simulink model "Cuk_cevirici"  (R2024b)
settings: Solver=ode23tb  StartTime=0.0  StopTime=0.2  RelTol=1e-3
libraries: spsMeanLib x10, spsSeriesRLCBranchLib x10, spsCurrentMeasurementLib x6, spsVoltageMeasurementLib x4, spsDCVoltageSourceLib x2, spsDiodeLib x2, spsGroundLib x2, spsIGBTLib x2, sps_lib x1
settings Model: Creator=m_pek  LastModifiedBy=m_pek

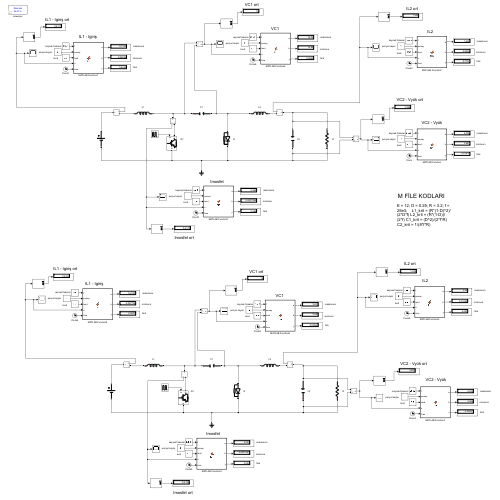
[thumbnail: Simulink's stored preview of the top-level diagram]
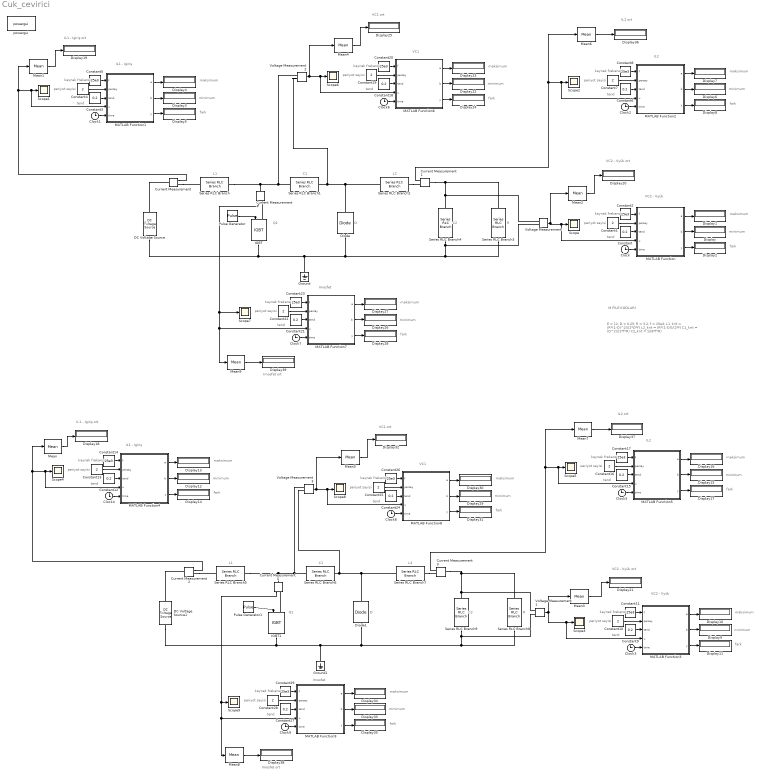
== system Cuk_cevirici ==
  note: M FİLE KODLARI
  note: E = 12; D = 0.25; R = 3.2; f = 25e3; L1_krit = (R*(1-D)^2)/(2*D*f) L2_krit = (R*(1-D))/(2*f) C1_krit = (D^2)/(2*f*R) C2_krit = 1/(8*f*R)
  note: L1
  note: C1
  note: L2
  note: C2
  note: R
  note: D
  note: Q1
  note: E
  note: minimum
  note: kaynak frekansi
  note: fark
  note: tend
  note: periyot sayisi
  note: maksimum
  note: minimum
  note: kaynak frekansi
  note: fark
  note: tend
  note: periyot sayisi
  note: maksimum
  note: minimum
  note: kaynak frekansi
  note: fark
  note: tend
  note: periyot sayisi
  note: maksimum
  note: L1
  note: C1
  note: L2
  note: C2
  note: R
  note: D
  note: Q1
  note: E
  note: minimum
  note: kaynak frekansi
  note: fark
  note: tend
  note: periyot sayisi
  note: maksimum
  note: minimum
  note: kaynak frekansi
  note: fark
  note: tend
  note: periyot sayisi
  note: maksimum
  note: minimum
  note: kaynak frekansi
  note: fark
  note: tend
  note: periyot sayisi
  note: maksimum
  note: VC2 - Vyük ort
  note: IL1 - Igiriş
  note: minimum
  note: kaynak frekansi
  note: fark
  note: tend
  note: periyot sayisi
  note: maksimum
  note: VC1 ort
  note: minimum
  note: kaynak frekansi
  note: fark
  note: tend
  note: periyot sayisi
  note: maksimum
  note: Imosfet
  note: IL1 - Igiriş ort
  note: IL1 - Igiriş ort
  note: IL2
  note: IL2
  note: minimum
  note: kaynak frekansi
  note: fark
  note: tend
  note: periyot sayisi
  note: maksimum
  note: VC1 ort
  note: minimum
  note: kaynak frekansi
  note: fark
  note: tend
  note: periyot sayisi
  note: maksimum
  note: Imosfet
  note: VC2 - Vyük ort
  note: IL2 ort
  note: VC1
  note: VC2 - Vyük
  note: IL2 ort
  note: VC2 - Vyük
  note: IL1 - Igiriş
  note: VC1
  note: Imosfet ort
  note: Imosfet ort
  Clock{,1..9} (10 alike) : Clock
      settings: Decimation=100
  Constant{,3,6,9,12,15,18,21,24,27} (10 alike) : Constant  Value=0.2  SampleTime=0
  Constant{1,4,7,10,13,16,19,22,25,28} (10 alike) : Constant  Value=2  SampleTime=0
  Constant{2,5,8,11,14,17,20,23,26,29} (10 alike) : Constant  Value=25e3  SampleTime=0
  Current Measurement{,1..5} (6 alike) : spsCurrentMeasurementLib/Current Measurement  PhasorSimulation=off  OutputType=Complex  PSBequivalent=0
  DC Voltage Source : spsDCVoltageSourceLib/DC Voltage Source  Amplitude=12  Measurements=None
  DC Voltage Source1 : spsDCVoltageSourceLib/DC Voltage Source  Amplitude=12  Measurements=None
  Diode : spsDiodeLib/Diode  Ron=0.0001  Lon=0  Vf=0.001  IC=0  UseSnubber=0  Rs=5000  Cs=250e-6  Measurements=off
  Diode1 : spsDiodeLib/Diode  Ron=0.0001  Lon=0  Vf=0.001  IC=0  UseSnubber=0  Rs=5000  Cs=250e-6  Measurements=off
  Display{,1..39} (40 alike) : Display
  Ground : spsGroundLib/Ground  LConnTagsString=a
  Ground1 : spsGroundLib/Ground  LConnTagsString=a
  IGBT : spsIGBTLib/IGBT  Ron=0.000001  Lon=0  Vf=0.00001  Tf=1e-6  Tt=2e-6  IC=0  Rs=1e5  Cs=inf  Measurements=off
  IGBT1 : spsIGBTLib/IGBT  Ron=0.000001  Lon=0  Vf=0.00001  Tf=1e-6  Tt=2e-6  IC=0  Rs=1e5  Cs=inf  Measurements=off
  MATLAB Function : MATLAB Function  TreatAsAtomicUnit=on
  MATLAB Function1 : MATLAB Function  TreatAsAtomicUnit=on
  MATLAB Function2 : MATLAB Function  TreatAsAtomicUnit=on
  MATLAB Function3 : MATLAB Function  TreatAsAtomicUnit=on
  MATLAB Function4 : MATLAB Function  TreatAsAtomicUnit=on
  MATLAB Function5 : MATLAB Function  TreatAsAtomicUnit=on
  MATLAB Function6 : MATLAB Function  TreatAsAtomicUnit=on
  MATLAB Function7 : MATLAB Function  TreatAsAtomicUnit=on
  MATLAB Function8 : MATLAB Function  TreatAsAtomicUnit=on
  MATLAB Function9 : MATLAB Function  TreatAsAtomicUnit=on
  Mean{,1..9} (10 alike) : spsMeanLib/Mean  Freq=25e3  Vinit=0  Ts=0
  Pulse Generator : DiscretePulseGenerator  PulseType=Time based  Period=0.00004  PulseWidth=25  VectorParams1D=off
  Pulse Generator1 : DiscretePulseGenerator  PulseType=Time based  Period=0.00004  PulseWidth=25  VectorParams1D=off
  Scope{,1..9} (10 alike) : Scope
  Series RLC Branch : spsSeriesRLCBranchLib/Series RLC Branch  LConnTagsString=__new0  RConnTagsString=__new0  BranchType=L  Resistance=1  Inductance=180e-6  SetiL0=off  InitialCurrent=0  Capacitance=1e-6  Setx0=off  InitialVoltage=0  Measurements=None
  Series RLC Branch1 : spsSeriesRLCBranchLib/Series RLC Branch  LConnTagsString=__new0  RConnTagsString=__new0  BranchType=C  Resistance=1  Inductance=1e-3  SetiL0=off  InitialCurrent=0  Capacitance=200e-6  Setx0=off  InitialVoltage=0  Measurements=None
  Series RLC Branch2 : spsSeriesRLCBranchLib/Series RLC Branch  LConnTagsString=__new0  RConnTagsString=__new0  BranchType=L  Resistance=1  Inductance=150e-6  SetiL0=off  InitialCurrent=0  Capacitance=1e-6  Setx0=off  InitialVoltage=0  Measurements=None
  Series RLC Branch3 : spsSeriesRLCBranchLib/Series RLC Branch  LConnTagsString=__new0  RConnTagsString=__new0  BranchType=R  Resistance=3.2  Inductance=1e-3  SetiL0=off  InitialCurrent=0  Capacitance=1e-6  Setx0=off  InitialVoltage=0  Measurements=None
  Series RLC Branch4 : spsSeriesRLCBranchLib/Series RLC Branch  LConnTagsString=__new0  RConnTagsString=__new0  BranchType=C  Resistance=1  Inductance=1e-3  SetiL0=off  InitialCurrent=0  Capacitance=220e-6  Setx0=off  InitialVoltage=0  Measurements=None
  Series RLC Branch5 : spsSeriesRLCBranchLib/Series RLC Branch  LConnTagsString=__new0  RConnTagsString=__new0  BranchType=L  Resistance=1  Inductance=1.4400e-04  SetiL0=off  InitialCurrent=0  Capacitance=1e-6  Setx0=off  InitialVoltage=0  Measurements=None
  Series RLC Branch6 : spsSeriesRLCBranchLib/Series RLC Branch  LConnTagsString=__new0  RConnTagsString=__new0  BranchType=C  Resistance=1  Inductance=1e-3  SetiL0=off  InitialCurrent=0  Capacitance=200e-6  Setx0=off  InitialVoltage=0  Measurements=None
  Series RLC Branch7 : spsSeriesRLCBranchLib/Series RLC Branch  LConnTagsString=__new0  RConnTagsString=__new0  BranchType=L  Resistance=1  Inductance=4.8000e-05  SetiL0=off  InitialCurrent=0  Capacitance=1e-6  Setx0=off  InitialVoltage=0  Measurements=None
  Series RLC Branch8 : spsSeriesRLCBranchLib/Series RLC Branch  LConnTagsString=__new0  RConnTagsString=__new0  BranchType=R  Resistance=3.2  Inductance=1e-3  SetiL0=off  InitialCurrent=0  Capacitance=1e-6  Setx0=off  InitialVoltage=0  Measurements=None
  Series RLC Branch9 : spsSeriesRLCBranchLib/Series RLC Branch  LConnTagsString=__new0  RConnTagsString=__new0  BranchType=C  Resistance=1  Inductance=1e-3  SetiL0=off  InitialCurrent=0  Capacitance=220e-6  Setx0=off  InitialVoltage=0  Measurements=None
  Voltage Measurement{,1..3} (4 alike) : spsVoltageMeasurementLib/Voltage Measurement  PhasorSimulation=off  OutputType=Complex  PSBequivalent=0
  powergui : sps_lib/powergui  Priority=1  SimulationMode=Discrete  SampleTime=50e-8  frequency=60  Iterations=50  frequencyindice=0  Pbase=100e6  ErrMax=1e-4  UnitsV=kV  UnitsW=MW  buscounter=0  FunctionMessages=off  echomessages=off  EnableUseOfTLC=off  CurrentSourceSwitches=off  DisableSnubberDevices=off  DisableRonSwitches=off  DisableVfSwitches=off  DisplayEquations=off  AutomaticDiscreteSolvers=off  SolverType=Tustin/Backward Euler (TBE)  Interpol=off  ExternalGateDelay=off  methode=off  Ts=100  x0status=zero  SPID=on  SwTol=0  HookPort=off  NonlinearTolerance=1e-4  nMaxIteration=100  ContinueOnMaxIteration=off  RestoreLinks=warning  ResistiveCurrentMeasurement=off  Frange=[0:2:500]  Ylog=off  Xlog=on  ShowGrid=off  save=off  variable=ZData  structure=0  ZoomFFT=off  StartTime=0.0  cycles=1  DisplayStyle=1  fundamental=60  FreqAxis=off  MaxFrequency=1000  frequencyindicesteady=1  RmsSteady=1  display=off
  wires:
  Pulse Generator/1 -> IGBT/1
  MATLAB Function/3(y) -> Display2/1
  MATLAB Function/2(b) -> Display/1
  Clock/1 -> MATLAB Function/5(time)
  Constant/1 -> MATLAB Function/3(tend)
  Constant2/1 -> MATLAB Function/1(f)
  MATLAB Function/1(a) -> Display1/1
  Constant1/1 -> MATLAB Function/2(persay)
  Constant4/1 -> MATLAB Function1/2(persay)
  MATLAB Function1/1(a) -> Display4/1
  Constant5/1 -> MATLAB Function1/1(f)
  Constant3/1 -> MATLAB Function1/3(tend)
  Current Measurement/1 -> Mean1/1, Scope1/1, MATLAB Function1/4(u)
  Clock1/1 -> MATLAB Function1/5(time)
  MATLAB Function1/2(b) -> Display3/1
  MATLAB Function1/3(y) -> Display5/1
  MATLAB Function2/3(y) -> Display8/1
  MATLAB Function2/2(b) -> Display6/1
  Clock2/1 -> MATLAB Function2/5(time)
  Current Measurement1/1 -> Mean6/1, MATLAB Function2/4(u), Scope2/1
  Constant6/1 -> MATLAB Function2/3(tend)
  Constant8/1 -> MATLAB Function2/1(f)
  MATLAB Function2/1(a) -> Display7/1
  Constant7/1 -> MATLAB Function2/2(persay)
  Constant16/1 -> MATLAB Function5/2(persay)
  MATLAB Function5/1(a) -> Display16/1
  Constant17/1 -> MATLAB Function5/1(f)
  Constant15/1 -> MATLAB Function5/3(tend)
  Clock5/1 -> MATLAB Function5/5(time)
  MATLAB Function5/2(b) -> Display15/1
  MATLAB Function5/3(y) -> Display17/1
  MATLAB Function4/3(y) -> Display14/1
  MATLAB Function4/2(b) -> Display12/1
  Clock4/1 -> MATLAB Function4/5(time)
  Current Measurement2/1 -> Mean/1, MATLAB Function4/4(u), Scope4/1
  Constant12/1 -> MATLAB Function4/3(tend)
  Constant14/1 -> MATLAB Function4/1(f)
  MATLAB Function4/1(a) -> Display13/1
  Constant13/1 -> MATLAB Function4/2(persay)
  Constant10/1 -> MATLAB Function3/2(persay)
  MATLAB Function3/1(a) -> Display10/1
  Constant11/1 -> MATLAB Function3/1(f)
  Constant9/1 -> MATLAB Function3/3(tend)
  Clock3/1 -> MATLAB Function3/5(time)
  MATLAB Function3/2(b) -> Display9/1
  MATLAB Function3/3(y) -> Display11/1
  Pulse Generator1/1 -> IGBT1/1
  Mean/1 -> Display18/1
  Mean1/1 -> Display19/1
  Mean2/1 -> Display20/1
  Voltage Measurement/1 -> MATLAB Function/4(u), Scope/1, Mean2/1
  Voltage Measurement1/1 -> Mean3/1, Scope3/1, MATLAB Function3/4(u)
  Mean3/1 -> Display21/1
  Voltage Measurement2/1 -> Scope6/1, MATLAB Function6/4(u), Mean4/1
  Mean4/1 -> Display25/1
  Constant19/1 -> MATLAB Function6/2(persay)
  MATLAB Function6/1(a) -> Display23/1
  Constant20/1 -> MATLAB Function6/1(f)
  Constant18/1 -> MATLAB Function6/3(tend)
  Clock6/1 -> MATLAB Function6/5(time)
  MATLAB Function6/2(b) -> Display22/1
  MATLAB Function6/3(y) -> Display24/1
  Constant22/1 -> MATLAB Function7/2(persay)
  MATLAB Function7/1(a) -> Display27/1
  Constant23/1 -> MATLAB Function7/1(f)
  Constant21/1 -> MATLAB Function7/3(tend)
  Clock7/1 -> MATLAB Function7/5(time)
  MATLAB Function7/2(b) -> Display26/1
  MATLAB Function7/3(y) -> Display28/1
  MATLAB Function8/3(y) -> Display31/1
  MATLAB Function8/2(b) -> Display29/1
  Clock8/1 -> MATLAB Function8/5(time)
  Constant24/1 -> MATLAB Function8/3(tend)
  Constant26/1 -> MATLAB Function8/1(f)
  MATLAB Function8/1(a) -> Display30/1
  Constant25/1 -> MATLAB Function8/2(persay)
  Mean5/1 -> Display32/1
  Voltage Measurement3/1 -> Mean5/1, MATLAB Function8/4(u), Scope8/1
  Current Measurement5/1 -> Mean8/1, MATLAB Function9/4(u), Scope9/1
  MATLAB Function9/3(y) -> Display35/1
  MATLAB Function9/2(b) -> Display33/1
  Clock9/1 -> MATLAB Function9/5(time)
  Constant27/1 -> MATLAB Function9/3(tend)
  Constant29/1 -> MATLAB Function9/1(f)
  MATLAB Function9/1(a) -> Display34/1
  Constant28/1 -> MATLAB Function9/2(persay)
  Mean6/1 -> Display36/1
  Mean7/1 -> Display37/1
  Current Measurement3/1 -> Mean7/1, Scope5/1, MATLAB Function5/4(u)
  Mean8/1 -> Display38/1
  Mean9/1 -> Display39/1
  Current Measurement4/1 -> Scope7/1, MATLAB Function7/4(u), Mean9/1
  connections:
  IGBT/LConn1 -- Current Measurement4/RConn1
  Series RLC Branch2/RConn1 -- Diode/LConn1 -- Voltage Measurement2/LConn2 -- Series RLC Branch1/RConn1
  Current Measurement1/LConn1 -- Voltage Measurement/LConn2 -- Series RLC Branch4/RConn1 -- Series RLC Branch3/RConn1
  DC Voltage Source/LConn1 -- Series RLC Branch4/LConn1 -- Voltage Measurement/LConn1 -- Series RLC Branch3/LConn1 -- Diode/RConn1 -- Ground/LConn1 -- IGBT/RConn1
  DC Voltage Source/RConn1 -- Current Measurement/LConn1
  Current Measurement/RConn1 -- Series RLC Branch/LConn1
  Series RLC Branch2/LConn1 -- Current Measurement1/RConn1
  Series RLC Branch5/RConn1 -- Voltage Measurement3/LConn1 -- Series RLC Branch6/LConn1 -- Current Measurement5/LConn1
  Series RLC Branch7/RConn1 -- Voltage Measurement3/LConn2 -- Series RLC Branch6/RConn1 -- Diode1/LConn1
  Series RLC Branch8/RConn1 -- Current Measurement3/LConn1 -- Voltage Measurement1/LConn2 -- Series RLC Branch9/RConn1
  DC Voltage Source1/LConn1 -- IGBT1/RConn1 -- Ground1/LConn1 -- Diode1/RConn1 -- Voltage Measurement1/LConn1 -- Series RLC Branch9/LConn1 -- Series RLC Branch8/LConn1
  Series RLC Branch7/LConn1 -- Current Measurement3/RConn1
  DC Voltage Source1/RConn1 -- Current Measurement2/LConn1
  Current Measurement2/RConn1 -- Series RLC Branch5/LConn1
  Current Measurement4/LConn1 -- Series RLC Branch/RConn1 -- Voltage Measurement2/LConn1 -- Series RLC Branch1/LConn1
  IGBT1/LConn1 -- Current Measurement5/RConn1

== matlab function Cuk_cevirici/MATLAB Function7 ==
  settings: updateMethod=DISCRETE  sampleTime=50e-8
  data: a output; b output; f input; persay input; tend input; u input; y output; time input
function [a,b,y] = fcn(f,persay,tend,u,time)
% persistent değişken; değişken değerini kalıcı olarak tutar ve direk atama
% yapılmadıkça değişmez. Normal değişkenler fonksiyonun her yenilenme 
% durumunda sıfırlanırken, persistent değişkeni, kalıcı olması sebebiyle,
% bir önceki değeri tutabilme yeteneğine sahiptir. 
% Bu da bize bir önceki değer ile güncel değerinizi karşılaştırma olanağı
% sunar.
a=1/0;b=0;
persistent enbuyuk;
persistent enkucuk;
persistent fark;
% Eğer persistent değişkenini en başta persistent enbuyuk = 0; olarak 
% tanımlarsak, sürekli 0 olarak kalacaktır. Aynı zamanda eğer bir ilk değer 
% vermezseniz "null" değerini taşıyacağından, if yapılarında hata
% verecektir. Bu hatadan kaçınmak için, isempty komutu ile persistent
% değişkenlerinin "null" olup olmadığını kontrol edilir ve ilk değer ataması
% yapılır. Bu değişkenler sadece  fonksiyon ilk kez çalıştığında
% null olacağı için(daha sonra sürekli gelen değeri tuttuğu yukarıda söylenmişti)
% başlangıçta, bir kereye mahsus olarak,  aşağıdaki if yapısı doğrulanacak 
% ve değişkenlere ilk değerler atanacaktır.
%
if (isempty(enkucuk) || isempty(enbuyuk))  
enkucuk = 1/0;   
enbuyuk = 0;
end
if (time>tend-(persay+1)*1/f) && (time<=tend) % Periyot ~= 0.01 // Son iki periyodu hesaplar.
    if u >= enbuyuk
        enbuyuk = u;
     end
    if u < enkucuk   
        enkucuk = u;
    end
end
fark = enbuyuk - enkucuk;
a=enbuyuk;
b=enkucuk;
y=fark;
end

== matlab function Cuk_cevirici/MATLAB Function8 ==
  settings: updateMethod=DISCRETE  sampleTime=50e-8
  data: a output; b output; f input; persay input; tend input; u input; y output; time input
function [a,b,y] = fcn(f,persay,tend,u,time)
% persistent değişken; değişken değerini kalıcı olarak tutar ve direk atama
% yapılmadıkça değişmez. Normal değişkenler fonksiyonun her yenilenme 
% durumunda sıfırlanırken, persistent değişkeni, kalıcı olması sebebiyle,
% bir önceki değeri tutabilme yeteneğine sahiptir. 
% Bu da bize bir önceki değer ile güncel değerinizi karşılaştırma olanağı
% sunar.
a=1/0;b=0;
persistent enbuyuk;
persistent enkucuk;
persistent fark;
% Eğer persistent değişkenini en başta persistent enbuyuk = 0; olarak 
% tanımlarsak, sürekli 0 olarak kalacaktır. Aynı zamanda eğer bir ilk değer 
% vermezseniz "null" değerini taşıyacağından, if yapılarında hata
% verecektir. Bu hatadan kaçınmak için, isempty komutu ile persistent
% değişkenlerinin "null" olup olmadığını kontrol edilir ve ilk değer ataması
% yapılır. Bu değişkenler sadece  fonksiyon ilk kez çalıştığında
% null olacağı için(daha sonra sürekli gelen değeri tuttuğu yukarıda söylenmişti)
% başlangıçta, bir kereye mahsus olarak,  aşağıdaki if yapısı doğrulanacak 
% ve değişkenlere ilk değerler atanacaktır.
%
if (isempty(enkucuk) || isempty(enbuyuk))  
enkucuk = 1/0;   
enbuyuk = 0;
end
if (time>tend-(persay+1)*1/f) && (time<=tend) % Periyot ~= 0.01 // Son iki periyodu hesaplar.
    if u >= enbuyuk
        enbuyuk = u;
     end
    if u < enkucuk   
        enkucuk = u;
    end
end
fark = enbuyuk - enkucuk;
a=enbuyuk;
b=enkucuk;
y=fark;
end

== matlab function Cuk_cevirici/MATLAB Function1 ==
  settings: updateMethod=DISCRETE  sampleTime=50e-8
  data: a output; b output; f input; persay input; tend input; u input; y output; time input
function [a,b,y] = fcn(f,persay,tend,u,time)
% persistent değişken; değişken değerini kalıcı olarak tutar ve direk atama
% yapılmadıkça değişmez. Normal değişkenler fonksiyonun her yenilenme 
% durumunda sıfırlanırken, persistent değişkeni, kalıcı olması sebebiyle,
% bir önceki değeri tutabilme yeteneğine sahiptir. 
% Bu da bize bir önceki değer ile güncel değerinizi karşılaştırma olanağı
% sunar.
a=1/0;b=0;
persistent enbuyuk;
persistent enkucuk;
persistent fark;
% Eğer persistent değişkenini en başta persistent enbuyuk = 0; olarak 
% tanımlarsak, sürekli 0 olarak kalacaktır. Aynı zamanda eğer bir ilk değer 
% vermezseniz "null" değerini taşıyacağından, if yapılarında hata
% verecektir. Bu hatadan kaçınmak için, isempty komutu ile persistent
% değişkenlerinin "null" olup olmadığını kontrol edilir ve ilk değer ataması
% yapılır. Bu değişkenler sadece  fonksiyon ilk kez çalıştığında
% null olacağı için(daha sonra sürekli gelen değeri tuttuğu yukarıda söylenmişti)
% başlangıçta, bir kereye mahsus olarak,  aşağıdaki if yapısı doğrulanacak 
% ve değişkenlere ilk değerler atanacaktır.
%
if (isempty(enkucuk) || isempty(enbuyuk))  
enkucuk = 1/0;   
enbuyuk = 0;
end
if (time>tend-(persay+1)*1/f) && (time<=tend) % Periyot ~= 0.01 // Son iki periyodu hesaplar.
    if u >= enbuyuk
        enbuyuk = u;
     end
    if u < enkucuk   
        enkucuk = u;
    end
end
fark = enbuyuk - enkucuk;
a=enbuyuk;
b=enkucuk;
y=fark;
end

== matlab function Cuk_cevirici/MATLAB Function9 ==
  settings: updateMethod=DISCRETE  sampleTime=50e-8
  data: a output; b output; f input; persay input; tend input; u input; y output; time input
function [a,b,y] = fcn(f,persay,tend,u,time)
% persistent değişken; değişken değerini kalıcı olarak tutar ve direk atama
% yapılmadıkça değişmez. Normal değişkenler fonksiyonun her yenilenme 
% durumunda sıfırlanırken, persistent değişkeni, kalıcı olması sebebiyle,
% bir önceki değeri tutabilme yeteneğine sahiptir. 
% Bu da bize bir önceki değer ile güncel değerinizi karşılaştırma olanağı
% sunar.
a=1/0;b=0;
persistent enbuyuk;
persistent enkucuk;
persistent fark;
% Eğer persistent değişkenini en başta persistent enbuyuk = 0; olarak 
% tanımlarsak, sürekli 0 olarak kalacaktır. Aynı zamanda eğer bir ilk değer 
% vermezseniz "null" değerini taşıyacağından, if yapılarında hata
% verecektir. Bu hatadan kaçınmak için, isempty komutu ile persistent
% değişkenlerinin "null" olup olmadığını kontrol edilir ve ilk değer ataması
% yapılır. Bu değişkenler sadece  fonksiyon ilk kez çalıştığında
% null olacağı için(daha sonra sürekli gelen değeri tuttuğu yukarıda söylenmişti)
% başlangıçta, bir kereye mahsus olarak,  aşağıdaki if yapısı doğrulanacak 
% ve değişkenlere ilk değerler atanacaktır.
%
if (isempty(enkucuk) || isempty(enbuyuk))  
enkucuk = 1/0;   
enbuyuk = 0;
end
if (time>tend-(persay+1)*1/f) && (time<=tend) % Periyot ~= 0.01 // Son iki periyodu hesaplar.
    if u >= enbuyuk
        enbuyuk = u;
     end
    if u < enkucuk   
        enkucuk = u;
    end
end
fark = enbuyuk - enkucuk;
a=enbuyuk;
b=enkucuk;
y=fark;
end

== matlab function Cuk_cevirici/MATLAB Function ==
  settings: updateMethod=DISCRETE  sampleTime=50e-8
  data: a output; b output; f input; persay input; tend input; u input; y output; time input
function [a,b,y] = fcn(f,persay,tend,u,time)
% persistent değişken; değişken değerini kalıcı olarak tutar ve direk atama
% yapılmadıkça değişmez. Normal değişkenler fonksiyonun her yenilenme 
% durumunda sıfırlanırken, persistent değişkeni, kalıcı olması sebebiyle,
% bir önceki değeri tutabilme yeteneğine sahiptir. 
% Bu da bize bir önceki değer ile güncel değerinizi karşılaştırma olanağı
% sunar.
a=1/0;b=0;
persistent enbuyuk;
persistent enkucuk;
persistent fark;
% Eğer persistent değişkenini en başta persistent enbuyuk = 0; olarak 
% tanımlarsak, sürekli 0 olarak kalacaktır. Aynı zamanda eğer bir ilk değer 
% vermezseniz "null" değerini taşıyacağından, if yapılarında hata
% verecektir. Bu hatadan kaçınmak için, isempty komutu ile persistent
% değişkenlerinin "null" olup olmadığını kontrol edilir ve ilk değer ataması
% yapılır. Bu değişkenler sadece  fonksiyon ilk kez çalıştığında
% null olacağı için(daha sonra sürekli gelen değeri tuttuğu yukarıda söylenmişti)
% başlangıçta, bir kereye mahsus olarak,  aşağıdaki if yapısı doğrulanacak 
% ve değişkenlere ilk değerler atanacaktır.
%
if (isempty(enkucuk) || isempty(enbuyuk))  
enkucuk = 1/0;   
enbuyuk = 0;
end
if (time>tend-(persay+1)*1/f) && (time<=tend) % Periyot ~= 0.01 // Son iki periyodu hesaplar.
    if u >= enbuyuk
        enbuyuk = u;
     end
    if u < enkucuk   
        enkucuk = u;
    end
end
fark = enbuyuk - enkucuk;
a=enbuyuk;
b=enkucuk;
y=fark;
end

== matlab function Cuk_cevirici/MATLAB Function2 ==
  settings: updateMethod=DISCRETE  sampleTime=50e-8
  data: a output; b output; f input; persay input; tend input; u input; y output; time input
function [a,b,y] = fcn(f,persay,tend,u,time)
% persistent değişken; değişken değerini kalıcı olarak tutar ve direk atama
% yapılmadıkça değişmez. Normal değişkenler fonksiyonun her yenilenme 
% durumunda sıfırlanırken, persistent değişkeni, kalıcı olması sebebiyle,
% bir önceki değeri tutabilme yeteneğine sahiptir. 
% Bu da bize bir önceki değer ile güncel değerinizi karşılaştırma olanağı
% sunar.
a=1/0;b=0;
persistent enbuyuk;
persistent enkucuk;
persistent fark;
% Eğer persistent değişkenini en başta persistent enbuyuk = 0; olarak 
% tanımlarsak, sürekli 0 olarak kalacaktır. Aynı zamanda eğer bir ilk değer 
% vermezseniz "null" değerini taşıyacağından, if yapılarında hata
% verecektir. Bu hatadan kaçınmak için, isempty komutu ile persistent
% değişkenlerinin "null" olup olmadığını kontrol edilir ve ilk değer ataması
% yapılır. Bu değişkenler sadece  fonksiyon ilk kez çalıştığında
% null olacağı için(daha sonra sürekli gelen değeri tuttuğu yukarıda söylenmişti)
% başlangıçta, bir kereye mahsus olarak,  aşağıdaki if yapısı doğrulanacak 
% ve değişkenlere ilk değerler atanacaktır.
%
if (isempty(enkucuk) || isempty(enbuyuk))  
enkucuk = 1/0;   
enbuyuk = 0;
end
if (time>tend-(persay+1)*1/f) && (time<=tend) % Periyot ~= 0.01 // Son iki periyodu hesaplar.
    if u >= enbuyuk
        enbuyuk = u;
     end
    if u < enkucuk   
        enkucuk = u;
    end
end
fark = enbuyuk - enkucuk;
a=enbuyuk;
b=enkucuk;
y=fark;
end

== matlab function Cuk_cevirici/MATLAB Function3 ==
  settings: updateMethod=DISCRETE  sampleTime=50e-8
  data: a output; b output; f input; persay input; tend input; u input; y output; time input
function [a,b,y] = fcn(f,persay,tend,u,time)
% persistent değişken; değişken değerini kalıcı olarak tutar ve direk atama
% yapılmadıkça değişmez. Normal değişkenler fonksiyonun her yenilenme 
% durumunda sıfırlanırken, persistent değişkeni, kalıcı olması sebebiyle,
% bir önceki değeri tutabilme yeteneğine sahiptir. 
% Bu da bize bir önceki değer ile güncel değerinizi karşılaştırma olanağı
% sunar.
a=1/0;b=0;
persistent enbuyuk;
persistent enkucuk;
persistent fark;
% Eğer persistent değişkenini en başta persistent enbuyuk = 0; olarak 
% tanımlarsak, sürekli 0 olarak kalacaktır. Aynı zamanda eğer bir ilk değer 
% vermezseniz "null" değerini taşıyacağından, if yapılarında hata
% verecektir. Bu hatadan kaçınmak için, isempty komutu ile persistent
% değişkenlerinin "null" olup olmadığını kontrol edilir ve ilk değer ataması
% yapılır. Bu değişkenler sadece  fonksiyon ilk kez çalıştığında
% null olacağı için(daha sonra sürekli gelen değeri tuttuğu yukarıda söylenmişti)
% başlangıçta, bir kereye mahsus olarak,  aşağıdaki if yapısı doğrulanacak 
% ve değişkenlere ilk değerler atanacaktır.
%
if (isempty(enkucuk) || isempty(enbuyuk))  
enkucuk = 1/0;   
enbuyuk = 0;
end
if (time>tend-(persay+1)*1/f) && (time<=tend) % Periyot ~= 0.01 // Son iki periyodu hesaplar.
    if u >= enbuyuk
        enbuyuk = u;
     end
    if u < enkucuk   
        enkucuk = u;
    end
end
fark = enbuyuk - enkucuk;
a=enbuyuk;
b=enkucuk;
y=fark;
end

== matlab function Cuk_cevirici/MATLAB Function4 ==
  settings: updateMethod=DISCRETE  sampleTime=50e-8
  data: a output; b output; f input; persay input; tend input; u input; y output; time input
function [a,b,y] = fcn(f,persay,tend,u,time)
% persistent değişken; değişken değerini kalıcı olarak tutar ve direk atama
% yapılmadıkça değişmez. Normal değişkenler fonksiyonun her yenilenme 
% durumunda sıfırlanırken, persistent değişkeni, kalıcı olması sebebiyle,
% bir önceki değeri tutabilme yeteneğine sahiptir. 
% Bu da bize bir önceki değer ile güncel değerinizi karşılaştırma olanağı
% sunar.
a=1/0;b=0;
persistent enbuyuk;
persistent enkucuk;
persistent fark;
% Eğer persistent değişkenini en başta persistent enbuyuk = 0; olarak 
% tanımlarsak, sürekli 0 olarak kalacaktır. Aynı zamanda eğer bir ilk değer 
% vermezseniz "null" değerini taşıyacağından, if yapılarında hata
% verecektir. Bu hatadan kaçınmak için, isempty komutu ile persistent
% değişkenlerinin "null" olup olmadığını kontrol edilir ve ilk değer ataması
% yapılır. Bu değişkenler sadece  fonksiyon ilk kez çalıştığında
% null olacağı için(daha sonra sürekli gelen değeri tuttuğu yukarıda söylenmişti)
% başlangıçta, bir kereye mahsus olarak,  aşağıdaki if yapısı doğrulanacak 
% ve değişkenlere ilk değerler atanacaktır.
%
if (isempty(enkucuk) || isempty(enbuyuk))  
enkucuk = 1/0;   
enbuyuk = 0;
end
if (time>tend-(persay+1)*1/f) && (time<=tend) % Periyot ~= 0.01 // Son iki periyodu hesaplar.
    if u >= enbuyuk
        enbuyuk = u;
     end
    if u < enkucuk   
        enkucuk = u;
    end
end
fark = enbuyuk - enkucuk;
a=enbuyuk;
b=enkucuk;
y=fark;
end

== matlab function Cuk_cevirici/MATLAB Function5 ==
  settings: updateMethod=DISCRETE  sampleTime=50e-8
  data: a output; b output; f input; persay input; tend input; u input; y output; time input
function [a,b,y] = fcn(f,persay,tend,u,time)
% persistent değişken; değişken değerini kalıcı olarak tutar ve direk atama
% yapılmadıkça değişmez. Normal değişkenler fonksiyonun her yenilenme 
% durumunda sıfırlanırken, persistent değişkeni, kalıcı olması sebebiyle,
% bir önceki değeri tutabilme yeteneğine sahiptir. 
% Bu da bize bir önceki değer ile güncel değerinizi karşılaştırma olanağı
% sunar.
a=1/0;b=0;
persistent enbuyuk;
persistent enkucuk;
persistent fark;
% Eğer persistent değişkenini en başta persistent enbuyuk = 0; olarak 
% tanımlarsak, sürekli 0 olarak kalacaktır. Aynı zamanda eğer bir ilk değer 
% vermezseniz "null" değerini taşıyacağından, if yapılarında hata
% verecektir. Bu hatadan kaçınmak için, isempty komutu ile persistent
% değişkenlerinin "null" olup olmadığını kontrol edilir ve ilk değer ataması
% yapılır. Bu değişkenler sadece  fonksiyon ilk kez çalıştığında
% null olacağı için(daha sonra sürekli gelen değeri tuttuğu yukarıda söylenmişti)
% başlangıçta, bir kereye mahsus olarak,  aşağıdaki if yapısı doğrulanacak 
% ve değişkenlere ilk değerler atanacaktır.
%
if (isempty(enkucuk) || isempty(enbuyuk))  
enkucuk = 1/0;   
enbuyuk = 0;
end
if (time>tend-(persay+1)*1/f) && (time<=tend) % Periyot ~= 0.01 // Son iki periyodu hesaplar.
    if u >= enbuyuk
        enbuyuk = u;
     end
    if u < enkucuk   
        enkucuk = u;
    end
end
fark = enbuyuk - enkucuk;
a=enbuyuk;
b=enkucuk;
y=fark;
end

== matlab function Cuk_cevirici/MATLAB Function6 ==
  settings: updateMethod=DISCRETE  sampleTime=50e-8
  data: a output; b output; f input; persay input; tend input; u input; y output; time input
function [a,b,y] = fcn(f,persay,tend,u,time)
% persistent değişken; değişken değerini kalıcı olarak tutar ve direk atama
% yapılmadıkça değişmez. Normal değişkenler fonksiyonun her yenilenme 
% durumunda sıfırlanırken, persistent değişkeni, kalıcı olması sebebiyle,
% bir önceki değeri tutabilme yeteneğine sahiptir. 
% Bu da bize bir önceki değer ile güncel değerinizi karşılaştırma olanağı
% sunar.
a=1/0;b=0;
persistent enbuyuk;
persistent enkucuk;
persistent fark;
% Eğer persistent değişkenini en başta persistent enbuyuk = 0; olarak 
% tanımlarsak, sürekli 0 olarak kalacaktır. Aynı zamanda eğer bir ilk değer 
% vermezseniz "null" değerini taşıyacağından, if yapılarında hata
% verecektir. Bu hatadan kaçınmak için, isempty komutu ile persistent
% değişkenlerinin "null" olup olmadığını kontrol edilir ve ilk değer ataması
% yapılır. Bu değişkenler sadece  fonksiyon ilk kez çalıştığında
% null olacağı için(daha sonra sürekli gelen değeri tuttuğu yukarıda söylenmişti)
% başlangıçta, bir kereye mahsus olarak,  aşağıdaki if yapısı doğrulanacak 
% ve değişkenlere ilk değerler atanacaktır.
%
if (isempty(enkucuk) || isempty(enbuyuk))  
enkucuk = 1/0;   
enbuyuk = 0;
end
if (time>tend-(persay+1)*1/f) && (time<=tend) % Periyot ~= 0.01 // Son iki periyodu hesaplar.
    if u >= enbuyuk
        enbuyuk = u;
     end
    if u < enkucuk   
        enkucuk = u;
    end
end
fark = enbuyuk - enkucuk;
a=enbuyuk;
b=enkucuk;
y=fark;
end
